simulink model "Lab2_AircraftEPS"  (Simulink 8.0)
settings: Solver=ode3  StartTime=0.0  StopTime=10  RelTol=1e-3
PreLoadFcn:
  | warning off
  | Ts=10e-6;
InitFcn:
  | warning off
  | Ts=10e-6;
undefined symbols (not defined in the file or in its folder): D1, Delta, sigbuilder_block
libraries: powerlib x91, sps_avr x4, powerlib_extras x4, checkVoltage x4
(part 2 of 2)

== system Lab2_AircraftEPS/TRU 28Vdc 4kW ==
  Ground1 : powerlib/Elements/Ground  LConnTagsString=a
  Ground2 : powerlib/Elements/Ground  LConnTagsString=a
  Ground4 : powerlib/Elements/Ground  LConnTagsString=a
  Series RLC Branch1 : powerlib/Elements/Series RLC Branch  LConnTagsString=__new0  RConnTagsString=__new0  BranchType=L  Resistance=[]  Inductance=2e-3  SetiL0=on  InitialCurrent=0  Capacitance=[]  Setx0=off  InitialVoltage=0  Measurements=Branch voltage and current
  Series RLC Branch2 : powerlib/Elements/Series RLC Branch  LConnTagsString=__new0  RConnTagsString=__new0  BranchType=C  Resistance=[]  Inductance=[]  SetiL0=off  InitialCurrent=0  Capacitance=1e-6  Setx0=off  InitialVoltage=0  Measurements=None
  Series RLC Branch4 : powerlib/Elements/Series RLC Branch  LConnTagsString=__new0  RConnTagsString=__new0  BranchType=L  Resistance=[]  Inductance=2e-3  SetiL0=off  InitialCurrent=0  Capacitance=[]  Setx0=off  InitialVoltage=0  Measurements=Branch voltage and current
  Three-Phase Transformer (Three Windings) : powerlib/Elements/Three-Phase Transformer (Three Windings)  Winding1Connection=Yn  UNITS=pu  NominalPower=[ 4200 , 400 ]  Winding1=[ 115 , 0.0002 , 0 ]  Winding2Connection=Delta (D1)  Winding2=[ 22 , 0.0002 , 0 ]  Winding3Connection=Delta (D1)  Winding3=[ 22 , 0.0002 , 0]  SetSaturation=off  Rm=500  Lm=500*10  Saturation=[ 0,0 ; 0.0024,1.2 ; 1.0,1.52 ]  Hysteresis=off  DataFile='hysteresis'  SetInitialFlux=off  InitialFluxes=[0.8 -0.8 0.7]  Measurements=None  MoreParameters=off  BreakLoop=off  DataType=off  TransfoNumber=0
  Universal Bridge : powerlib/Power Electronics/Universal Bridge  Arms=3  SnubberResistance=1e3  SnubberCapacitance=1e-6  Device=Diodes  Ron=1e-3  Lon=0  ForwardVoltages="[  0  0  ]"  ForwardVoltage=0.8  GTOparameters=[ 10e-6 , 20e-6 ]  IGBTparameters=[ 1e-6 , 2e-6 ]  Measurements=None  Measurements_2=None  converterType=Rectifier
  Universal Bridge1 : powerlib/Power Electronics/Universal Bridge  Arms=3  SnubberResistance=1e3  SnubberCapacitance=1e-6  Device=Diodes  Ron=1e-3  Lon=0  ForwardVoltages="[  0  0  ]"  ForwardVoltage=0.8  GTOparameters=[ 10e-6 , 20e-6 ]  IGBTparameters=[ 1e-6 , 2e-6 ]  Measurements=None  Measurements_2=None  converterType=Rectifier
  A : PMIOPort  Port=1  Side=Left
  B : PMIOPort  Port=2  Side=Left
  + : PMIOPort  Port=3  Side=Right
  C : PMIOPort  Port=4  Side=Left
  connections:
  Ground2/LConn1 -- Series RLC Branch2/RConn1
  Ground1/LConn1 -- Universal Bridge/RConn2 -- Universal Bridge1/RConn2
  Three-Phase Transformer (Three Windings)/RConn1 -- Universal Bridge/LConn1
  Three-Phase Transformer (Three Windings)/RConn2 -- Universal Bridge/LConn2
  Three-Phase Transformer (Three Windings)/RConn3 -- Universal Bridge/LConn3
  A/RConn1 -- Three-Phase Transformer (Three Windings)/LConn1
  B/RConn1 -- Three-Phase Transformer (Three Windings)/LConn2
  C/RConn1 -- Three-Phase Transformer (Three Windings)/LConn3
  Ground4/LConn1 -- Three-Phase Transformer (Three Windings)/LConn4
  Series RLC Branch1/LConn1 -- Universal Bridge/RConn1
  Series RLC Branch2/LConn1 -- Series RLC Branch1/RConn1 -- +/RConn1 -- Series RLC Branch4/LConn1
  Three-Phase Transformer (Three Windings)/RConn4 -- Universal Bridge1/LConn1
  Three-Phase Transformer (Three Windings)/RConn5 -- Universal Bridge1/LConn2
  Three-Phase Transformer (Three Windings)/RConn6 -- Universal Bridge1/LConn3
  Universal Bridge1/RConn1 -- Series RLC Branch4/RConn1

== system Lab2_AircraftEPS/TRU 28Vdc 4kW3 ==
  Ground1 : powerlib/Elements/Ground  LConnTagsString=a
  Ground2 : powerlib/Elements/Ground  LConnTagsString=a
  Ground4 : powerlib/Elements/Ground  LConnTagsString=a
  Series RLC Branch1 : powerlib/Elements/Series RLC Branch  LConnTagsString=__new0  RConnTagsString=__new0  BranchType=L  Resistance=[]  Inductance=2e-3  SetiL0=on  InitialCurrent=0  Capacitance=[]  Setx0=off  InitialVoltage=0  Measurements=Branch voltage and current
  Series RLC Branch2 : powerlib/Elements/Series RLC Branch  LConnTagsString=__new0  RConnTagsString=__new0  BranchType=C  Resistance=[]  Inductance=[]  SetiL0=off  InitialCurrent=0  Capacitance=1e-6  Setx0=off  InitialVoltage=0  Measurements=None
  Series RLC Branch4 : powerlib/Elements/Series RLC Branch  LConnTagsString=__new0  RConnTagsString=__new0  BranchType=L  Resistance=[]  Inductance=2e-3  SetiL0=off  InitialCurrent=0  Capacitance=[]  Setx0=off  InitialVoltage=0  Measurements=Branch voltage and current
  Three-Phase Transformer (Three Windings) : powerlib/Elements/Three-Phase Transformer (Three Windings)  Winding1Connection=Yn  UNITS=pu  NominalPower=[ 4200 , 400 ]  Winding1=[ 115 , 0.0002 , 0 ]  Winding2Connection=Delta (D1)  Winding2=[ 22 , 0.0002 , 0 ]  Winding3Connection=Delta (D1)  Winding3=[ 22 , 0.0002 , 0]  SetSaturation=off  Rm=500  Lm=500*10  Saturation=[ 0,0 ; 0.0024,1.2 ; 1.0,1.52 ]  Hysteresis=off  DataFile='hysteresis'  SetInitialFlux=off  InitialFluxes=[0.8 -0.8 0.7]  Measurements=None  MoreParameters=off  BreakLoop=off  DataType=off  TransfoNumber=0
  Universal Bridge : powerlib/Power Electronics/Universal Bridge  Arms=3  SnubberResistance=1e3  SnubberCapacitance=1e-6  Device=Diodes  Ron=1e-3  Lon=0  ForwardVoltages="[  0  0  ]"  ForwardVoltage=0.8  GTOparameters=[ 10e-6 , 20e-6 ]  IGBTparameters=[ 1e-6 , 2e-6 ]  Measurements=None  Measurements_2=None  converterType=Rectifier
  Universal Bridge1 : powerlib/Power Electronics/Universal Bridge  Arms=3  SnubberResistance=1e3  SnubberCapacitance=1e-6  Device=Diodes  Ron=1e-3  Lon=0  ForwardVoltages="[  0  0  ]"  ForwardVoltage=0.8  GTOparameters=[ 10e-6 , 20e-6 ]  IGBTparameters=[ 1e-6 , 2e-6 ]  Measurements=None  Measurements_2=None  converterType=Rectifier
  A : PMIOPort  Port=1  Side=Left
  B : PMIOPort  Port=2  Side=Left
  + : PMIOPort  Port=3  Side=Right
  C : PMIOPort  Port=4  Side=Left
  connections:
  Ground2/LConn1 -- Series RLC Branch2/RConn1
  Ground1/LConn1 -- Universal Bridge/RConn2 -- Universal Bridge1/RConn2
  Three-Phase Transformer (Three Windings)/RConn1 -- Universal Bridge/LConn1
  Three-Phase Transformer (Three Windings)/RConn2 -- Universal Bridge/LConn2
  Three-Phase Transformer (Three Windings)/RConn3 -- Universal Bridge/LConn3
  A/RConn1 -- Three-Phase Transformer (Three Windings)/LConn1
  B/RConn1 -- Three-Phase Transformer (Three Windings)/LConn2
  C/RConn1 -- Three-Phase Transformer (Three Windings)/LConn3
  Ground4/LConn1 -- Three-Phase Transformer (Three Windings)/LConn4
  Series RLC Branch1/LConn1 -- Universal Bridge/RConn1
  Series RLC Branch2/LConn1 -- Series RLC Branch1/RConn1 -- +/RConn1 -- Series RLC Branch4/LConn1
  Three-Phase Transformer (Three Windings)/RConn4 -- Universal Bridge1/LConn1
  Three-Phase Transformer (Three Windings)/RConn5 -- Universal Bridge1/LConn2
  Three-Phase Transformer (Three Windings)/RConn6 -- Universal Bridge1/LConn3
  Universal Bridge1/RConn1 -- Series RLC Branch4/RConn1

== system Lab2_AircraftEPS/APU1/Fault Contactor ==
  Fault : Inport
  In1 : Inport  Port=2
  Constant : Constant  Value=0
  Switch : Switch  Threshold=0.5
  out : Outport
  wires:
  Fault/1 -> Switch/2
  Constant/1 -> Switch/3
  In1/1 -> Switch/1
  Switch/1 -> out/1

== system Lab2_AircraftEPS/APU1/Feedback measurements &  main contactor ==
  note: Primary Distribution
  GLC control : Inport
  Contactor : Subsystem
  P.O.R  and CTA : powerlib/Measurements/Three-Phase V-I Measurement  VoltageMeasurement=phase-to-phase  SetLabelV=off  LabelV=Vabc  Vpu=off  VpuLL=off  CurrentMeasurement=yes  SetLabelI=off  LabelI=Iabc  Ipu=off  Pbase=100e6  Vbase=500e3  OutputType=Complex  PhasorSimulation=off  PSBequivalent=0
  parasitic resistive load : powerlib/Elements/Three-Phase Series RLC Load  LConnTagsString=A|B|C  Configuration=Y (grounded)  NominalVoltage=115  NominalFrequency=400  ActivePower=5000  InductivePower=0  CapacitivePower=0  Measurements=None  LoadType=constant Z
  in_a : PMIOPort  Port=1  Side=Left
  in_b : PMIOPort  Port=2  Side=Left
  in_c : PMIOPort  Port=3  Side=Left
  out_a : PMIOPort  Port=4  Side=Right
  out_b : PMIOPort  Port=5  Side=Right
  out_c : PMIOPort  Port=6  Side=Right
  Vabc : Outport
  Iabc : Outport  Port=2
  wires:
  GLC control/1 -> Contactor/1(com)
  P.O.R  and CTA/1 -> Vabc/1
  P.O.R  and CTA/2 -> Iabc/1
  connections:
  in_a/RConn1 -- P.O.R  and CTA/LConn1 -- parasitic resistive load/LConn1
  in_b/RConn1 -- P.O.R  and CTA/LConn2 -- parasitic resistive load/LConn2
  in_c/RConn1 -- P.O.R  and CTA/LConn3 -- parasitic resistive load/LConn3
  P.O.R  and CTA/RConn1 -- Contactor/LConn1
  P.O.R  and CTA/RConn2 -- Contactor/LConn2
  P.O.R  and CTA/RConn3 -- Contactor/LConn3
  Contactor/RConn1 -- out_a/RConn1
  out_b/RConn1 -- Contactor/RConn2
  Contactor/RConn3 -- out_c/RConn1

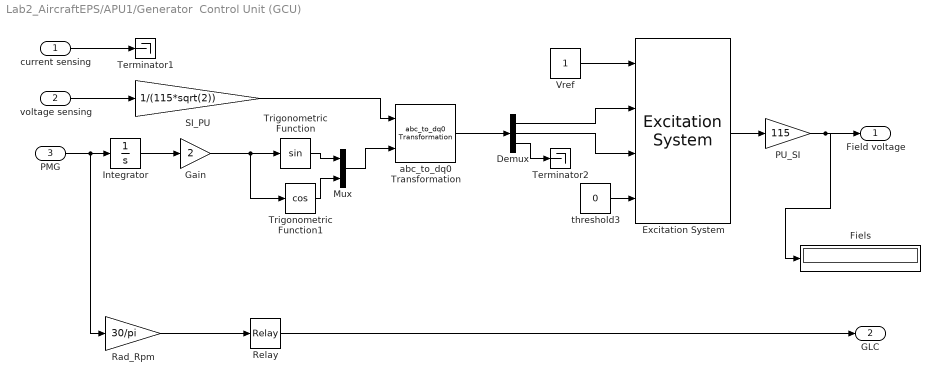
== system Lab2_AircraftEPS/APU1/Generator  Control Unit (GCU) ==
  current sensing : Inport
  voltage sensing : Inport  Port=2
  PMG : Inport  Port=3
  Demux : Demux  Outputs=3
  Excitation System : sps_avr/Excitation System   tr=20e-3  reg=[ 300, 0.001 ]  exc=[ 1, 0 ]  tgr=[ 0, 0 ]  damp=[ 0.001, 0.1 ]  sat=[ 0, 0 ]  lim=[ -2, 2, 0 ]  v0=[1 0]
  Fiels : Display
      settings: SampleTime=1e-2
  Gain : Gain  Gain=2
  Integrator : Integrator
  Mux : Mux  Inputs=2
  PU_SI : Gain  Gain=115
  Rad_Rpm : Gain  Gain=30/pi
  Relay : Relay  OnSwitchValue=9000  OffSwitchValue=8900
  SI_PU : Gain  Gain=1/(115*sqrt(2))
  Terminator1 : Terminator
  Terminator2 : Terminator
  Trigonometric Function : Trigonometry
  Trigonometric Function1 : Trigonometry  Operator=cos
  Vref : Constant
  abc_to_dq0 Transformation : powerlib_extras/Measurements/abc_to_dq0 Transformation
  threshold3 : Constant  Value=0
  Field voltage : Outport
  GLC : Outport  Port=2
  wires:
  Relay/1 -> GLC/1
  Demux/3 -> Terminator2/1
  current sensing/1 -> Terminator1/1
  threshold3/1 -> Excitation System/4
  Vref/1 -> Excitation System/1
  Rad_Rpm/1 -> Relay/1
  PU_SI/1 -> Field voltage/1, Fiels/1
  Excitation System/1 -> PU_SI/1
  SI_PU/1 -> abc_to_dq0 Transformation/1
  Demux/2 -> Excitation System/3
  Demux/1 -> Excitation System/2
  abc_to_dq0 Transformation/1 -> Demux/1
  Mux/1 -> abc_to_dq0 Transformation/2
  Trigonometric Function1/1 -> Mux/2
  Trigonometric Function/1 -> Mux/1
  Gain/1 -> Trigonometric Function1/1, Trigonometric Function/1
  Integrator/1 -> Gain/1
  voltage sensing/1 -> SI_PU/1
  PMG/1 -> Rad_Rpm/1, Integrator/1

== system Lab2_AircraftEPS/APU1/Mechanical engine (turbine) ==
  Demux : Demux  Tag=STV Demux  Outputs=1
  FromWs : FromWorkspace  Tag=STV FromWs  VariableName=tuvar  SampleTime=0  SigBuilderData=DataTag0  VnvData=DataTag1
      SigBuilderData=|
      | common.afterFinalStr = 'Extrapolate'
      | common.sampleTime = 0
      | dataSet.timeRange = [0 10]
      | dataSet.name = 'Group 1'
      | sbobj.Groups.Name = 'Group 1'
      | sbobj.Groups.Signals.Name = 'Signal 1'
      | sbobj.Groups.Signals.XData = [0 0.2 0.4 0.5 1 2 3 4.5 6 10]
      | sbobj.Groups.Signals.YData = [15000 15000 15000 15000 15000 15000 15000 15000 15000 15000]
  Signal 1 : Outport  Tag=STV Outport
  wires:
  FromWs/1 -> Demux/1
  Demux/1 -> Signal 1/1

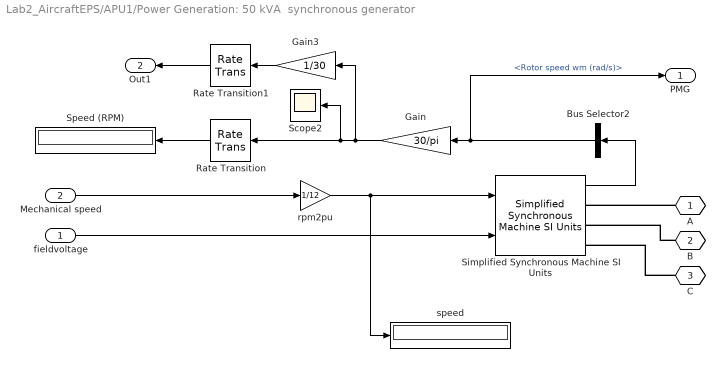
== system Lab2_AircraftEPS/APU1/Power Generation: 50 kVA  synchronous generator ==
  fieldvoltage : Inport
  Mechanical speed : Inport  Port=2
  Bus Selector2 : BusSelector  OutputSignals=Rotor speed wm (rad/s)
  Gain : Gain  Gain=30/pi
  Gain3 : Gain  Gain=1/30
  Rate Transition : RateTransition  OutPortSampleTimeOpt=Inherit  OutPortSampleTime=Ts
  Rate Transition1 : RateTransition  OutPortSampleTimeOpt=Inherit  OutPortSampleTime=Ts
  Scope2 : Scope
      settings: TimeRange=1  YMin=13545  YMax=13575  SaveName=ScopeData3  Decimation=100  SampleTime=1e-3
  Simplified Synchronous Machine SI Units : powerlib/Machines/Simplified Synchronous Machine SI Units  ConnectionType=3-wire Y  MechanicalLoad=Speed w  NominalParameters=[50e3 115 400]  Mechanical=[0.02 0 2]  InternalRL="[0.0204  0.08104e-3]"  InitialConditions=[-99,0 0,0,0 0,0,0]  Units=1  LoadFlowParameters=[1 0 0 0 0]  TsPowergui=0  TsBlock=-1  BusType=PV  Pref=0  Qref=0  Qmin=-inf  Qmax=+inf  PLF=0  QLF=0
  Speed (RPM) : Display
      settings: SampleTime=1e-2
  rpm2pu : Gain  Gain=1/12
  speed : Display
      settings: SampleTime=1e-2
  A : PMIOPort  Tag=PMCPort  Port=1  Side=Right
  B : PMIOPort  Tag=PMCPort  Port=2  Side=Right
  C : PMIOPort  Tag=PMCPort  Port=3  Side=Right
  PMG : Outport
  Out1 : Outport  Port=2
  wires:
  Simplified Synchronous Machine SI Units/1 -> Bus Selector2/1
  fieldvoltage/1 -> Simplified Synchronous Machine SI Units/2
  Bus Selector2/1 -> Gain/1, PMG/1  "<Rotor speed wm (rad/s)>"
  Gain/1 -> Gain3/1, Scope2/1, Rate Transition/1
  Gain3/1 -> Rate Transition1/1
  Mechanical speed/1 -> rpm2pu/1
  rpm2pu/1 -> Simplified Synchronous Machine SI Units/1, speed/1
  Rate Transition/1 -> Speed (RPM)/1
  Rate Transition1/1 -> Out1/1
  connections:
  A/RConn1 -- Simplified Synchronous Machine SI Units/RConn1
  B/RConn1 -- Simplified Synchronous Machine SI Units/RConn2
  C/RConn1 -- Simplified Synchronous Machine SI Units/RConn3

== system Lab2_AircraftEPS/APU1/Sensor ==
  Three Phase  Measurement : powerlib/Measurements/Three-Phase V-I Measurement  VoltageMeasurement=phase-to-phase  SetLabelV=off  LabelV=Vabc  Vpu=off  VpuLL=off  CurrentMeasurement=yes  SetLabelI=off  LabelI=Iabc  Ipu=off  Pbase=100e6  Vbase=500e3  OutputType=Complex  PhasorSimulation=off  PSBequivalent=0
  parasitic  load : powerlib/Elements/Three-Phase Series RLC Load  LConnTagsString=A|B|C  Configuration=Y (grounded)  NominalVoltage=115  NominalFrequency=400  ActivePower=5000  InductivePower=0  CapacitivePower=0  Measurements=None  LoadType=constant Z
  A : PMIOPort  Port=1  Side=Left
  B : PMIOPort  Port=2  Side=Left
  a : PMIOPort  Port=3  Side=Right
  b : PMIOPort  Port=4  Side=Right
  C : PMIOPort  Port=5  Side=Left
  c : PMIOPort  Port=6  Side=Right
  Vabc : Outport
  Iabc : Outport  Port=2
  wires:
  Three Phase  Measurement/1 -> Vabc/1
  Three Phase  Measurement/2 -> Iabc/1
  connections:
  A/RConn1 -- Three Phase  Measurement/LConn1 -- parasitic  load/LConn1
  B/RConn1 -- Three Phase  Measurement/LConn2 -- parasitic  load/LConn2
  C/RConn1 -- Three Phase  Measurement/LConn3 -- parasitic  load/LConn3
  a/RConn1 -- Three Phase  Measurement/RConn1
  b/RConn1 -- Three Phase  Measurement/RConn2
  c/RConn1 -- Three Phase  Measurement/RConn3

== system Lab2_AircraftEPS/APU2/Fault Contactor ==
  Fault : Inport
  In1 : Inport  Port=2
  Constant : Constant  Value=0
  Switch : Switch  Threshold=0.5
  out : Outport
  wires:
  Fault/1 -> Switch/2
  Constant/1 -> Switch/3
  In1/1 -> Switch/1
  Switch/1 -> out/1

== system Lab2_AircraftEPS/APU2/Feedback measurements &  main contactor ==
  note: Primary Distribution
  GLC control : Inport
  Contactor : Subsystem
  P.O.R  and CTA : powerlib/Measurements/Three-Phase V-I Measurement  VoltageMeasurement=phase-to-phase  SetLabelV=off  LabelV=Vabc  Vpu=off  VpuLL=off  CurrentMeasurement=yes  SetLabelI=off  LabelI=Iabc  Ipu=off  Pbase=100e6  Vbase=500e3  OutputType=Complex  PhasorSimulation=off  PSBequivalent=0
  parasitic resistive load : powerlib/Elements/Three-Phase Series RLC Load  LConnTagsString=A|B|C  Configuration=Y (grounded)  NominalVoltage=200  NominalFrequency=400  ActivePower=5000  InductivePower=0  CapacitivePower=0  Measurements=None  LoadType=constant Z
  in_a : PMIOPort  Port=1  Side=Left
  in_b : PMIOPort  Port=2  Side=Left
  in_c : PMIOPort  Port=3  Side=Left
  out_a : PMIOPort  Port=4  Side=Right
  out_b : PMIOPort  Port=5  Side=Right
  out_c : PMIOPort  Port=6  Side=Right
  Vabc : Outport
  Iabc : Outport  Port=2
  wires:
  GLC control/1 -> Contactor/1(com)
  P.O.R  and CTA/1 -> Vabc/1
  P.O.R  and CTA/2 -> Iabc/1
  connections:
  in_a/RConn1 -- P.O.R  and CTA/LConn1 -- parasitic resistive load/LConn1
  in_b/RConn1 -- P.O.R  and CTA/LConn2 -- parasitic resistive load/LConn2
  in_c/RConn1 -- P.O.R  and CTA/LConn3 -- parasitic resistive load/LConn3
  P.O.R  and CTA/RConn1 -- Contactor/LConn1
  P.O.R  and CTA/RConn2 -- Contactor/LConn2
  P.O.R  and CTA/RConn3 -- Contactor/LConn3
  Contactor/RConn1 -- out_a/RConn1
  out_b/RConn1 -- Contactor/RConn2
  Contactor/RConn3 -- out_c/RConn1

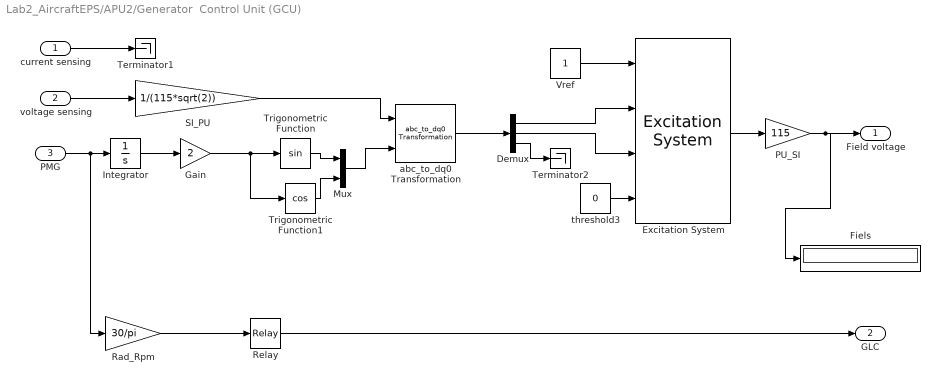
== system Lab2_AircraftEPS/APU2/Generator  Control Unit (GCU) ==
  current sensing : Inport
  voltage sensing : Inport  Port=2
  PMG : Inport  Port=3
  Demux : Demux  Outputs=3
  Excitation System : sps_avr/Excitation System   tr=20e-3  reg=[ 300, 0.001 ]  exc=[ 1, 0 ]  tgr=[ 0, 0 ]  damp=[ 0.001, 0.1 ]  sat=[ 0, 0 ]  lim=[ -2, 2, 0 ]  v0=[1 0]
  Fiels : Display
      settings: SampleTime=1e-2
  Gain : Gain  Gain=2
  Integrator : Integrator
  Mux : Mux  Inputs=2
  PU_SI : Gain  Gain=115
  Rad_Rpm : Gain  Gain=30/pi
  Relay : Relay  OnSwitchValue=9000  OffSwitchValue=8900
  SI_PU : Gain  Gain=1/(115*sqrt(2))
  Terminator1 : Terminator
  Terminator2 : Terminator
  Trigonometric Function : Trigonometry
  Trigonometric Function1 : Trigonometry  Operator=cos
  Vref : Constant
  abc_to_dq0 Transformation : powerlib_extras/Measurements/abc_to_dq0 Transformation
  threshold3 : Constant  Value=0
  Field voltage : Outport
  GLC : Outport  Port=2
  wires:
  Relay/1 -> GLC/1
  Demux/3 -> Terminator2/1
  current sensing/1 -> Terminator1/1
  threshold3/1 -> Excitation System/4
  Vref/1 -> Excitation System/1
  Rad_Rpm/1 -> Relay/1
  PU_SI/1 -> Field voltage/1, Fiels/1
  Excitation System/1 -> PU_SI/1
  SI_PU/1 -> abc_to_dq0 Transformation/1
  Demux/2 -> Excitation System/3
  Demux/1 -> Excitation System/2
  abc_to_dq0 Transformation/1 -> Demux/1
  Mux/1 -> abc_to_dq0 Transformation/2
  Trigonometric Function1/1 -> Mux/2
  Trigonometric Function/1 -> Mux/1
  Gain/1 -> Trigonometric Function1/1, Trigonometric Function/1
  Integrator/1 -> Gain/1
  voltage sensing/1 -> SI_PU/1
  PMG/1 -> Rad_Rpm/1, Integrator/1

== system Lab2_AircraftEPS/APU2/Mechanical engine (turbine) ==
  Demux : Demux  Tag=STV Demux  Outputs=1
  FromWs : FromWorkspace  Tag=STV FromWs  VariableName=tuvar  SampleTime=0  SigBuilderData=DataTag2  VnvData=DataTag3
      SigBuilderData=|
      | common.afterFinalStr = 'Extrapolate'
      | common.sampleTime = 0
      | dataSet.timeRange = [0 10]
      | dataSet.name = 'Group 1'
      | sbobj.Groups.Name = 'Group 1'
      | sbobj.Groups.Signals.Name = 'Signal 1'
      | sbobj.Groups.Signals.XData = [0 0.2 0.4 0.5 1 2 3 4.5 6 10]
      | sbobj.Groups.Signals.YData = [15000 15000 15000 15000 15000 15000 15000 15000 15000 15000]
  Signal 1 : Outport  Tag=STV Outport
  wires:
  FromWs/1 -> Demux/1
  Demux/1 -> Signal 1/1

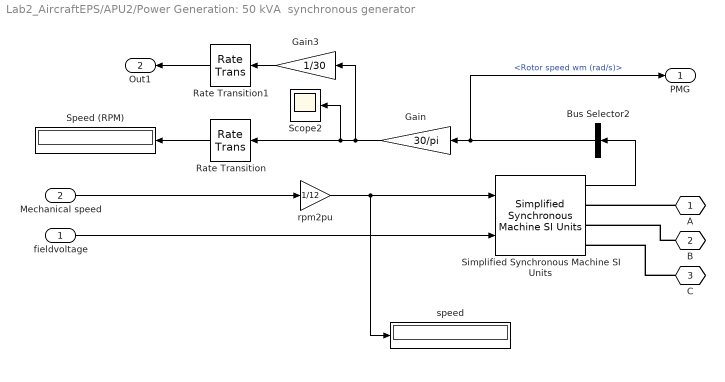
== system Lab2_AircraftEPS/APU2/Power Generation: 50 kVA  synchronous generator ==
  fieldvoltage : Inport
  Mechanical speed : Inport  Port=2
  Bus Selector2 : BusSelector  OutputSignals=Rotor speed wm (rad/s)
  Gain : Gain  Gain=30/pi
  Gain3 : Gain  Gain=1/30
  Rate Transition : RateTransition  OutPortSampleTimeOpt=Inherit  OutPortSampleTime=Ts
  Rate Transition1 : RateTransition  OutPortSampleTimeOpt=Inherit  OutPortSampleTime=Ts
  Scope2 : Scope
      settings: TimeRange=1  YMin=13545  YMax=13575  SaveName=ScopeData3  Decimation=100  SampleTime=1e-3
  Simplified Synchronous Machine SI Units : powerlib/Machines/Simplified Synchronous Machine SI Units  ConnectionType=3-wire Y  MechanicalLoad=Speed w  NominalParameters=[50e3 115 400]  Mechanical=[0.02 0 2]  InternalRL="[0.0204  0.08104e-3]"  InitialConditions=[-99,0 0,0,0 0,0,0]  Units=1  LoadFlowParameters=[1 0 0 0 0]  TsPowergui=0  TsBlock=-1  BusType=PV  Pref=0  Qref=0  Qmin=-inf  Qmax=+inf  PLF=0  QLF=0
  Speed (RPM) : Display
      settings: SampleTime=1e-2
  rpm2pu : Gain  Gain=1/12
  speed : Display
      settings: SampleTime=1e-2
  A : PMIOPort  Tag=PMCPort  Port=1  Side=Right
  B : PMIOPort  Tag=PMCPort  Port=2  Side=Right
  C : PMIOPort  Tag=PMCPort  Port=3  Side=Right
  PMG : Outport
  Out1 : Outport  Port=2
  wires:
  Simplified Synchronous Machine SI Units/1 -> Bus Selector2/1
  fieldvoltage/1 -> Simplified Synchronous Machine SI Units/2
  Bus Selector2/1 -> Gain/1, PMG/1  "<Rotor speed wm (rad/s)>"
  Gain/1 -> Gain3/1, Scope2/1, Rate Transition/1
  Gain3/1 -> Rate Transition1/1
  Mechanical speed/1 -> rpm2pu/1
  rpm2pu/1 -> Simplified Synchronous Machine SI Units/1, speed/1
  Rate Transition/1 -> Speed (RPM)/1
  Rate Transition1/1 -> Out1/1
  connections:
  A/RConn1 -- Simplified Synchronous Machine SI Units/RConn1
  B/RConn1 -- Simplified Synchronous Machine SI Units/RConn2
  C/RConn1 -- Simplified Synchronous Machine SI Units/RConn3

== system Lab2_AircraftEPS/APU2/Sensor ==
  Three Phase  Measurement : powerlib/Measurements/Three-Phase V-I Measurement  VoltageMeasurement=phase-to-phase  SetLabelV=off  LabelV=Vabc  Vpu=off  VpuLL=off  CurrentMeasurement=yes  SetLabelI=off  LabelI=Iabc  Ipu=off  Pbase=100e6  Vbase=500e3  OutputType=Complex  PhasorSimulation=off  PSBequivalent=0
  parasitic  load : powerlib/Elements/Three-Phase Series RLC Load  LConnTagsString=A|B|C  Configuration=Y (grounded)  NominalVoltage=115  NominalFrequency=400  ActivePower=5000  InductivePower=0  CapacitivePower=0  Measurements=None  LoadType=constant Z
  A : PMIOPort  Port=1  Side=Left
  B : PMIOPort  Port=2  Side=Left
  a : PMIOPort  Port=3  Side=Right
  b : PMIOPort  Port=4  Side=Right
  C : PMIOPort  Port=5  Side=Left
  c : PMIOPort  Port=6  Side=Right
  Vabc : Outport
  Iabc : Outport  Port=2
  wires:
  Three Phase  Measurement/1 -> Vabc/1
  Three Phase  Measurement/2 -> Iabc/1
  connections:
  A/RConn1 -- Three Phase  Measurement/LConn1 -- parasitic  load/LConn1
  B/RConn1 -- Three Phase  Measurement/LConn2 -- parasitic  load/LConn2
  C/RConn1 -- Three Phase  Measurement/LConn3 -- parasitic  load/LConn3
  a/RConn1 -- Three Phase  Measurement/RConn1
  b/RConn1 -- Three Phase  Measurement/RConn2
  c/RConn1 -- Three Phase  Measurement/RConn3

== system Lab2_AircraftEPS/B1/Contactor ==
  com : Inport
  Ideal Switch : powerlib/Power Electronics/Ideal Switch  Ron=0.001  Lon=0  IC=0  Rs=1e3  Cs=inf  Measurements=off
  Ideal Switch1 : powerlib/Power Electronics/Ideal Switch  Ron=0.001  Lon=0  IC=0  Rs=1e3  Cs=inf  Measurements=off
  Ideal Switch2 : powerlib/Power Electronics/Ideal Switch  Ron=0.001  Lon=0  IC=0  Rs=1e3  Cs=inf  Measurements=off
  A : PMIOPort  Port=1  Side=Left
  a : PMIOPort  Port=2  Side=Right
  B : PMIOPort  Port=3  Side=Left
  b : PMIOPort  Port=4  Side=Right
  C : PMIOPort  Port=5  Side=Left
  c : PMIOPort  Port=6  Side=Right
  wires:
  com/1 -> Ideal Switch/1, Ideal Switch2/1, Ideal Switch1/1
  connections:
  A/RConn1 -- Ideal Switch/LConn1
  a/RConn1 -- Ideal Switch/RConn1
  B/RConn1 -- Ideal Switch1/LConn1
  b/RConn1 -- Ideal Switch1/RConn1
  C/RConn1 -- Ideal Switch2/LConn1
  c/RConn1 -- Ideal Switch2/RConn1

== system Lab2_AircraftEPS/B10/Contactor ==
  com : Inport
  Ideal Switch : powerlib/Power Electronics/Ideal Switch  Ron=0.001  Lon=0  IC=0  Rs=1e3  Cs=inf  Measurements=off
  A : PMIOPort  Port=1  Side=Left
  a : PMIOPort  Port=2  Side=Right
  wires:
  com/1 -> Ideal Switch/1
  connections:
  A/RConn1 -- Ideal Switch/LConn1
  a/RConn1 -- Ideal Switch/RConn1

== system Lab2_AircraftEPS/B11/Contactor ==
  com : Inport
  Ideal Switch : powerlib/Power Electronics/Ideal Switch  Ron=0.001  Lon=0  IC=0  Rs=1e3  Cs=inf  Measurements=off
  A : PMIOPort  Port=1  Side=Left
  a : PMIOPort  Port=2  Side=Right
  wires:
  com/1 -> Ideal Switch/1
  connections:
  A/RConn1 -- Ideal Switch/LConn1
  a/RConn1 -- Ideal Switch/RConn1

== system Lab2_AircraftEPS/B12/Contactor ==
  com : Inport
  Ideal Switch : powerlib/Power Electronics/Ideal Switch  Ron=0.001  Lon=0  IC=0  Rs=1e3  Cs=inf  Measurements=off
  A : PMIOPort  Port=1  Side=Left
  a : PMIOPort  Port=2  Side=Right
  wires:
  com/1 -> Ideal Switch/1
  connections:
  A/RConn1 -- Ideal Switch/LConn1
  a/RConn1 -- Ideal Switch/RConn1

== system Lab2_AircraftEPS/B2/Contactor ==
  com : Inport
  Ideal Switch : powerlib/Power Electronics/Ideal Switch  Ron=0.001  Lon=0  IC=0  Rs=1e3  Cs=inf  Measurements=off
  Ideal Switch1 : powerlib/Power Electronics/Ideal Switch  Ron=0.001  Lon=0  IC=0  Rs=1e3  Cs=inf  Measurements=off
  Ideal Switch2 : powerlib/Power Electronics/Ideal Switch  Ron=0.001  Lon=0  IC=0  Rs=1e3  Cs=inf  Measurements=off
  A : PMIOPort  Port=1  Side=Left
  a : PMIOPort  Port=2  Side=Right
  B : PMIOPort  Port=3  Side=Left
  b : PMIOPort  Port=4  Side=Right
  C : PMIOPort  Port=5  Side=Left
  c : PMIOPort  Port=6  Side=Right
  wires:
  com/1 -> Ideal Switch/1, Ideal Switch2/1, Ideal Switch1/1
  connections:
  A/RConn1 -- Ideal Switch/LConn1
  a/RConn1 -- Ideal Switch/RConn1
  B/RConn1 -- Ideal Switch1/LConn1
  b/RConn1 -- Ideal Switch1/RConn1
  C/RConn1 -- Ideal Switch2/LConn1
  c/RConn1 -- Ideal Switch2/RConn1

== system Lab2_AircraftEPS/B3/Contactor ==
  com : Inport
  Ideal Switch : powerlib/Power Electronics/Ideal Switch  Ron=0.001  Lon=0  IC=0  Rs=1e3  Cs=inf  Measurements=off
  Ideal Switch1 : powerlib/Power Electronics/Ideal Switch  Ron=0.001  Lon=0  IC=0  Rs=1e3  Cs=inf  Measurements=off
  Ideal Switch2 : powerlib/Power Electronics/Ideal Switch  Ron=0.001  Lon=0  IC=0  Rs=1e3  Cs=inf  Measurements=off
  A : PMIOPort  Port=1  Side=Left
  a : PMIOPort  Port=2  Side=Right
  B : PMIOPort  Port=3  Side=Left
  b : PMIOPort  Port=4  Side=Right
  C : PMIOPort  Port=5  Side=Left
  c : PMIOPort  Port=6  Side=Right
  wires:
  com/1 -> Ideal Switch/1, Ideal Switch2/1, Ideal Switch1/1
  connections:
  A/RConn1 -- Ideal Switch/LConn1
  a/RConn1 -- Ideal Switch/RConn1
  B/RConn1 -- Ideal Switch1/LConn1
  b/RConn1 -- Ideal Switch1/RConn1
  C/RConn1 -- Ideal Switch2/LConn1
  c/RConn1 -- Ideal Switch2/RConn1

== system Lab2_AircraftEPS/B4/Contactor ==
  com : Inport
  Ideal Switch : powerlib/Power Electronics/Ideal Switch  Ron=0.001  Lon=0  IC=0  Rs=1e3  Cs=inf  Measurements=off
  Ideal Switch1 : powerlib/Power Electronics/Ideal Switch  Ron=0.001  Lon=0  IC=0  Rs=1e3  Cs=inf  Measurements=off
  Ideal Switch2 : powerlib/Power Electronics/Ideal Switch  Ron=0.001  Lon=0  IC=0  Rs=1e3  Cs=inf  Measurements=off
  A : PMIOPort  Port=1  Side=Left
  a : PMIOPort  Port=2  Side=Right
  B : PMIOPort  Port=3  Side=Left
  b : PMIOPort  Port=4  Side=Right
  C : PMIOPort  Port=5  Side=Left
  c : PMIOPort  Port=6  Side=Right
  wires:
  com/1 -> Ideal Switch/1, Ideal Switch2/1, Ideal Switch1/1
  connections:
  A/RConn1 -- Ideal Switch/LConn1
  a/RConn1 -- Ideal Switch/RConn1
  B/RConn1 -- Ideal Switch1/LConn1
  b/RConn1 -- Ideal Switch1/RConn1
  C/RConn1 -- Ideal Switch2/LConn1
  c/RConn1 -- Ideal Switch2/RConn1

== system Lab2_AircraftEPS/B5/Contactor ==
  com : Inport
  Ideal Switch : powerlib/Power Electronics/Ideal Switch  Ron=0.001  Lon=0  IC=0  Rs=1e3  Cs=inf  Measurements=off
  Ideal Switch1 : powerlib/Power Electronics/Ideal Switch  Ron=0.001  Lon=0  IC=0  Rs=1e3  Cs=inf  Measurements=off
  Ideal Switch2 : powerlib/Power Electronics/Ideal Switch  Ron=0.001  Lon=0  IC=0  Rs=1e3  Cs=inf  Measurements=off
  A : PMIOPort  Port=1  Side=Left
  a : PMIOPort  Port=2  Side=Right
  B : PMIOPort  Port=3  Side=Left
  b : PMIOPort  Port=4  Side=Right
  C : PMIOPort  Port=5  Side=Left
  c : PMIOPort  Port=6  Side=Right
  wires:
  com/1 -> Ideal Switch/1, Ideal Switch2/1, Ideal Switch1/1
  connections:
  A/RConn1 -- Ideal Switch/LConn1
  a/RConn1 -- Ideal Switch/RConn1
  B/RConn1 -- Ideal Switch1/LConn1
  b/RConn1 -- Ideal Switch1/RConn1
  C/RConn1 -- Ideal Switch2/LConn1
  c/RConn1 -- Ideal Switch2/RConn1

== system Lab2_AircraftEPS/B6/Contactor ==
  com : Inport
  Ideal Switch : powerlib/Power Electronics/Ideal Switch  Ron=0.001  Lon=0  IC=0  Rs=1e3  Cs=inf  Measurements=off
  Ideal Switch1 : powerlib/Power Electronics/Ideal Switch  Ron=0.001  Lon=0  IC=0  Rs=1e3  Cs=inf  Measurements=off
  Ideal Switch2 : powerlib/Power Electronics/Ideal Switch  Ron=0.001  Lon=0  IC=0  Rs=1e3  Cs=inf  Measurements=off
  A : PMIOPort  Port=1  Side=Left
  a : PMIOPort  Port=2  Side=Right
  B : PMIOPort  Port=3  Side=Left
  b : PMIOPort  Port=4  Side=Right
  C : PMIOPort  Port=5  Side=Left
  c : PMIOPort  Port=6  Side=Right
  wires:
  com/1 -> Ideal Switch/1, Ideal Switch2/1, Ideal Switch1/1
  connections:
  A/RConn1 -- Ideal Switch/LConn1
  a/RConn1 -- Ideal Switch/RConn1
  B/RConn1 -- Ideal Switch1/LConn1
  b/RConn1 -- Ideal Switch1/RConn1
  C/RConn1 -- Ideal Switch2/LConn1
  c/RConn1 -- Ideal Switch2/RConn1

== system Lab2_AircraftEPS/B7/Contactor ==
  com : Inport
  Ideal Switch : powerlib/Power Electronics/Ideal Switch  Ron=0.001  Lon=0  IC=0  Rs=1e3  Cs=inf  Measurements=off
  Ideal Switch1 : powerlib/Power Electronics/Ideal Switch  Ron=0.001  Lon=0  IC=0  Rs=1e3  Cs=inf  Measurements=off
  Ideal Switch2 : powerlib/Power Electronics/Ideal Switch  Ron=0.001  Lon=0  IC=0  Rs=1e3  Cs=inf  Measurements=off
  A : PMIOPort  Port=1  Side=Left
  a : PMIOPort  Port=2  Side=Right
  B : PMIOPort  Port=3  Side=Left
  b : PMIOPort  Port=4  Side=Right
  C : PMIOPort  Port=5  Side=Left
  c : PMIOPort  Port=6  Side=Right
  wires:
  com/1 -> Ideal Switch/1, Ideal Switch2/1, Ideal Switch1/1
  connections:
  A/RConn1 -- Ideal Switch/LConn1
  a/RConn1 -- Ideal Switch/RConn1
  B/RConn1 -- Ideal Switch1/LConn1
  b/RConn1 -- Ideal Switch1/RConn1
  C/RConn1 -- Ideal Switch2/LConn1
  c/RConn1 -- Ideal Switch2/RConn1

== system Lab2_AircraftEPS/B8/Contactor ==
  com : Inport
  Ideal Switch : powerlib/Power Electronics/Ideal Switch  Ron=0.001  Lon=0  IC=0  Rs=1e3  Cs=inf  Measurements=off
  Ideal Switch1 : powerlib/Power Electronics/Ideal Switch  Ron=0.001  Lon=0  IC=0  Rs=1e3  Cs=inf  Measurements=off
  Ideal Switch2 : powerlib/Power Electronics/Ideal Switch  Ron=0.001  Lon=0  IC=0  Rs=1e3  Cs=inf  Measurements=off
  A : PMIOPort  Port=1  Side=Left
  a : PMIOPort  Port=2  Side=Right
  B : PMIOPort  Port=3  Side=Left
  b : PMIOPort  Port=4  Side=Right
  C : PMIOPort  Port=5  Side=Left
  c : PMIOPort  Port=6  Side=Right
  wires:
  com/1 -> Ideal Switch/1, Ideal Switch2/1, Ideal Switch1/1
  connections:
  A/RConn1 -- Ideal Switch/LConn1
  a/RConn1 -- Ideal Switch/RConn1
  B/RConn1 -- Ideal Switch1/LConn1
  b/RConn1 -- Ideal Switch1/RConn1
  C/RConn1 -- Ideal Switch2/LConn1
  c/RConn1 -- Ideal Switch2/RConn1

== system Lab2_AircraftEPS/B9/Contactor ==
  com : Inport
  Ideal Switch : powerlib/Power Electronics/Ideal Switch  Ron=0.001  Lon=0  IC=0  Rs=1e3  Cs=inf  Measurements=off
  A : PMIOPort  Port=1  Side=Left
  a : PMIOPort  Port=2  Side=Right
  wires:
  com/1 -> Ideal Switch/1
  connections:
  A/RConn1 -- Ideal Switch/LConn1
  a/RConn1 -- Ideal Switch/RConn1

== system Lab2_AircraftEPS/BPCU/UNUSED -  Load Management ==
  Constant : Constant
  Constant1 : Constant  Value=0
  B7 : Outport
  B8 : Outport  Port=2
  B9 : Outport  Port=3
  B10 : Outport  Port=4
  B11 : Outport  Port=5
  B12 : Outport  Port=6
  wires:
  Constant/1 -> B10/1, B9/1, B8/1, B7/1
  Constant1/1 -> B11/1, B12/1

== system Lab2_AircraftEPS/Left Engine HV/Fault Contactor ==
  Fault : Inport
  In1 : Inport  Port=2
  Constant : Constant  Value=0
  Switch : Switch  Threshold=0.5
  out : Outport
  wires:
  Fault/1 -> Switch/2
  Constant/1 -> Switch/3
  In1/1 -> Switch/1
  Switch/1 -> out/1

== system Lab2_AircraftEPS/Left Engine HV/Feedback measurements &  main contactor ==
  note: Primary Distribution
  GLC control : Inport
  Contactor : Subsystem
  P.O.R  and CTA : powerlib/Measurements/Three-Phase V-I Measurement  VoltageMeasurement=phase-to-phase  SetLabelV=off  LabelV=Vabc  Vpu=off  VpuLL=off  CurrentMeasurement=yes  SetLabelI=off  LabelI=Iabc  Ipu=off  Pbase=100e6  Vbase=500e3  OutputType=Complex  PhasorSimulation=off  PSBequivalent=0
  parasitic resistive load : powerlib/Elements/Three-Phase Series RLC Load  LConnTagsString=A|B|C  Configuration=Y (grounded)  NominalVoltage=115  NominalFrequency=400  ActivePower=5000  InductivePower=0  CapacitivePower=0  Measurements=None  LoadType=constant Z
  in_a : PMIOPort  Port=1  Side=Left
  in_b : PMIOPort  Port=2  Side=Left
  in_c : PMIOPort  Port=3  Side=Left
  out_a : PMIOPort  Port=4  Side=Right
  out_b : PMIOPort  Port=5  Side=Right
  out_c : PMIOPort  Port=6  Side=Right
  Vabc : Outport
  Iabc : Outport  Port=2
  wires:
  GLC control/1 -> Contactor/1(com)
  P.O.R  and CTA/1 -> Vabc/1
  P.O.R  and CTA/2 -> Iabc/1
  connections:
  in_a/RConn1 -- P.O.R  and CTA/LConn1 -- parasitic resistive load/LConn1
  in_b/RConn1 -- P.O.R  and CTA/LConn2 -- parasitic resistive load/LConn2
  in_c/RConn1 -- P.O.R  and CTA/LConn3 -- parasitic resistive load/LConn3
  P.O.R  and CTA/RConn1 -- Contactor/LConn1
  P.O.R  and CTA/RConn2 -- Contactor/LConn2
  P.O.R  and CTA/RConn3 -- Contactor/LConn3
  Contactor/RConn1 -- out_a/RConn1
  out_b/RConn1 -- Contactor/RConn2
  Contactor/RConn3 -- out_c/RConn1

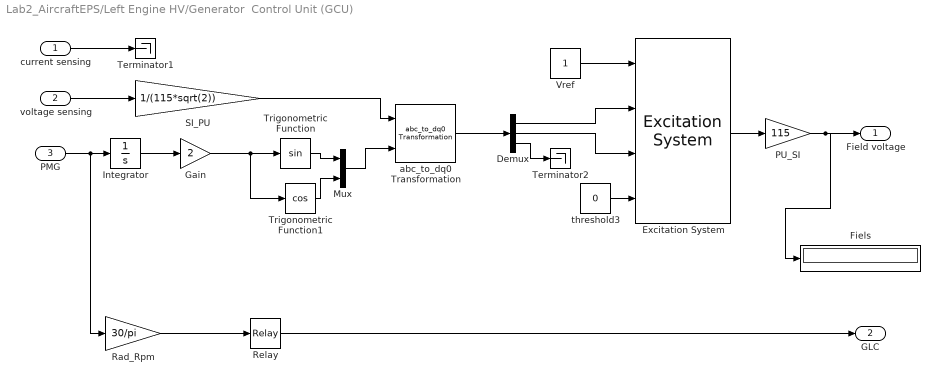
== system Lab2_AircraftEPS/Left Engine HV/Generator  Control Unit (GCU) ==
  current sensing : Inport
  voltage sensing : Inport  Port=2
  PMG : Inport  Port=3
  Demux : Demux  Outputs=3
  Excitation System : sps_avr/Excitation System   tr=20e-3  reg=[ 300, 0.001 ]  exc=[ 1, 0 ]  tgr=[ 0, 0 ]  damp=[ 0.001, 0.1 ]  sat=[ 0, 0 ]  lim=[ -2, 2, 0 ]  v0=[1 0]
  Fiels : Display
      settings: SampleTime=1e-2
  Gain : Gain  Gain=2
  Integrator : Integrator
  Mux : Mux  Inputs=2
  PU_SI : Gain  Gain=115
  Rad_Rpm : Gain  Gain=30/pi
  Relay : Relay  OnSwitchValue=9000  OffSwitchValue=8900
  SI_PU : Gain  Gain=1/(115*sqrt(2))
  Terminator1 : Terminator
  Terminator2 : Terminator
  Trigonometric Function : Trigonometry
  Trigonometric Function1 : Trigonometry  Operator=cos
  Vref : Constant
  abc_to_dq0 Transformation : powerlib_extras/Measurements/abc_to_dq0 Transformation
  threshold3 : Constant  Value=0
  Field voltage : Outport
  GLC : Outport  Port=2
  wires:
  Relay/1 -> GLC/1
  Demux/3 -> Terminator2/1
  current sensing/1 -> Terminator1/1
  threshold3/1 -> Excitation System/4
  Vref/1 -> Excitation System/1
  Rad_Rpm/1 -> Relay/1
  PU_SI/1 -> Field voltage/1, Fiels/1
  Excitation System/1 -> PU_SI/1
  SI_PU/1 -> abc_to_dq0 Transformation/1
  Demux/2 -> Excitation System/3
  Demux/1 -> Excitation System/2
  abc_to_dq0 Transformation/1 -> Demux/1
  Mux/1 -> abc_to_dq0 Transformation/2
  Trigonometric Function1/1 -> Mux/2
  Trigonometric Function/1 -> Mux/1
  Gain/1 -> Trigonometric Function1/1, Trigonometric Function/1
  Integrator/1 -> Gain/1
  voltage sensing/1 -> SI_PU/1
  PMG/1 -> Rad_Rpm/1, Integrator/1

== system Lab2_AircraftEPS/Left Engine HV/Mechanical engine (turbine) ==
  Demux : Demux  Tag=STV Demux  Outputs=1
  FromWs : FromWorkspace  Tag=STV FromWs  VariableName=tuvar  SampleTime=0  SigBuilderData=DataTag4  VnvData=DataTag5
      SigBuilderData=|
      | common.afterFinalStr = 'Extrapolate'
      | common.sampleTime = 0
      | dataSet.timeRange = [0 10]
      | dataSet.name = 'Group 1'
      | sbobj.Groups.Name = 'Group 1'
      | sbobj.Groups.Signals.Name = 'Signal 1'
      | sbobj.Groups.Signals.XData = [0 0.2 0.4 0.5 1 2 3 4.5 6 10]
      | sbobj.Groups.Signals.YData = [15000 15000 15000 15000 15000 15000 15000 15000 15000 15000]
  Signal 1 : Outport  Tag=STV Outport
  wires:
  FromWs/1 -> Demux/1
  Demux/1 -> Signal 1/1

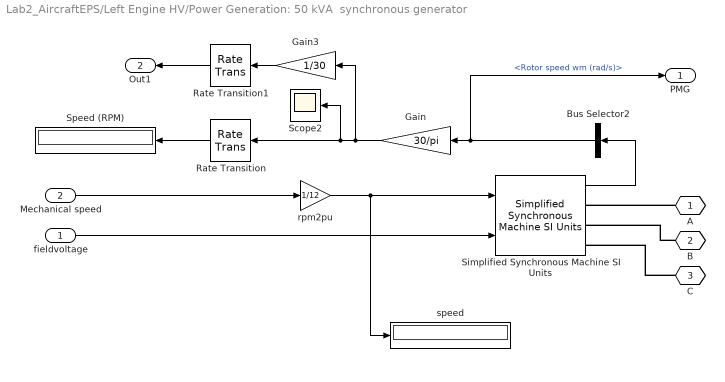
== system Lab2_AircraftEPS/Left Engine HV/Power Generation: 50 kVA  synchronous generator ==
  fieldvoltage : Inport
  Mechanical speed : Inport  Port=2
  Bus Selector2 : BusSelector  OutputSignals=Rotor speed wm (rad/s)
  Gain : Gain  Gain=30/pi
  Gain3 : Gain  Gain=1/30
  Rate Transition : RateTransition  OutPortSampleTimeOpt=Inherit  OutPortSampleTime=Ts
  Rate Transition1 : RateTransition  OutPortSampleTimeOpt=Inherit  OutPortSampleTime=Ts
  Scope2 : Scope
      settings: TimeRange=1  YMin=13545  YMax=13575  SaveName=ScopeData3  Decimation=100  SampleTime=1e-3
  Simplified Synchronous Machine SI Units : powerlib/Machines/Simplified Synchronous Machine SI Units  ConnectionType=3-wire Y  MechanicalLoad=Speed w  NominalParameters=[50e3 115 400]  Mechanical=[0.02 0 2]  InternalRL="[0.0204  0.08104e-3]"  InitialConditions=[-99,0 0,0,0 0,0,0]  Units=1  LoadFlowParameters=[1 0 0 0 0]  TsPowergui=0  TsBlock=-1  BusType=PV  Pref=0  Qref=0  Qmin=-inf  Qmax=+inf  PLF=0  QLF=0
  Speed (RPM) : Display
      settings: SampleTime=1e-2
  rpm2pu : Gain  Gain=1/12
  speed : Display
      settings: SampleTime=1e-2
  A : PMIOPort  Tag=PMCPort  Port=1  Side=Right
  B : PMIOPort  Tag=PMCPort  Port=2  Side=Right
  C : PMIOPort  Tag=PMCPort  Port=3  Side=Right
  PMG : Outport
  Out1 : Outport  Port=2
  wires:
  Simplified Synchronous Machine SI Units/1 -> Bus Selector2/1
  fieldvoltage/1 -> Simplified Synchronous Machine SI Units/2
  Bus Selector2/1 -> Gain/1, PMG/1  "<Rotor speed wm (rad/s)>"
  Gain/1 -> Gain3/1, Scope2/1, Rate Transition/1
  Gain3/1 -> Rate Transition1/1
  Mechanical speed/1 -> rpm2pu/1
  rpm2pu/1 -> Simplified Synchronous Machine SI Units/1, speed/1
  Rate Transition/1 -> Speed (RPM)/1
  Rate Transition1/1 -> Out1/1
  connections:
  A/RConn1 -- Simplified Synchronous Machine SI Units/RConn1
  B/RConn1 -- Simplified Synchronous Machine SI Units/RConn2
  C/RConn1 -- Simplified Synchronous Machine SI Units/RConn3

== system Lab2_AircraftEPS/Left Engine HV/Sensor ==
  Three Phase  Measurement : powerlib/Measurements/Three-Phase V-I Measurement  VoltageMeasurement=phase-to-phase  SetLabelV=off  LabelV=Vabc  Vpu=off  VpuLL=off  CurrentMeasurement=yes  SetLabelI=off  LabelI=Iabc  Ipu=off  Pbase=100e6  Vbase=500e3  OutputType=Complex  PhasorSimulation=off  PSBequivalent=0
  parasitic  load : powerlib/Elements/Three-Phase Series RLC Load  LConnTagsString=A|B|C  Configuration=Y (grounded)  NominalVoltage=115  NominalFrequency=400  ActivePower=5000  InductivePower=0  CapacitivePower=0  Measurements=None  LoadType=constant Z
  A : PMIOPort  Port=1  Side=Left
  B : PMIOPort  Port=2  Side=Left
  a : PMIOPort  Port=3  Side=Right
  b : PMIOPort  Port=4  Side=Right
  C : PMIOPort  Port=5  Side=Left
  c : PMIOPort  Port=6  Side=Right
  Vabc : Outport
  Iabc : Outport  Port=2
  wires:
  Three Phase  Measurement/1 -> Vabc/1
  Three Phase  Measurement/2 -> Iabc/1
  connections:
  A/RConn1 -- Three Phase  Measurement/LConn1 -- parasitic  load/LConn1
  B/RConn1 -- Three Phase  Measurement/LConn2 -- parasitic  load/LConn2
  C/RConn1 -- Three Phase  Measurement/LConn3 -- parasitic  load/LConn3
  a/RConn1 -- Three Phase  Measurement/RConn1
  b/RConn1 -- Three Phase  Measurement/RConn2
  c/RConn1 -- Three Phase  Measurement/RConn3

== system Lab2_AircraftEPS/Right Engine HV/Fault Contactor ==
  Fault : Inport
  In1 : Inport  Port=2
  Constant : Constant  Value=0
  Switch : Switch  Threshold=0.5
  out : Outport
  wires:
  Fault/1 -> Switch/2
  Constant/1 -> Switch/3
  In1/1 -> Switch/1
  Switch/1 -> out/1

== system Lab2_AircraftEPS/Right Engine HV/Feedback measurements &  main contactor ==
  note: Primary Distribution
  GLC control : Inport
  Contactor : Subsystem
  P.O.R  and CTA : powerlib/Measurements/Three-Phase V-I Measurement  VoltageMeasurement=phase-to-phase  SetLabelV=off  LabelV=Vabc  Vpu=off  VpuLL=off  CurrentMeasurement=yes  SetLabelI=off  LabelI=Iabc  Ipu=off  Pbase=100e6  Vbase=500e3  OutputType=Complex  PhasorSimulation=off  PSBequivalent=0
  parasitic resistive load : powerlib/Elements/Three-Phase Series RLC Load  LConnTagsString=A|B|C  Configuration=Y (grounded)  NominalVoltage=115  NominalFrequency=400  ActivePower=5000  InductivePower=0  CapacitivePower=0  Measurements=None  LoadType=constant Z
  in_a : PMIOPort  Port=1  Side=Left
  in_b : PMIOPort  Port=2  Side=Left
  in_c : PMIOPort  Port=3  Side=Left
  out_a : PMIOPort  Port=4  Side=Right
  out_b : PMIOPort  Port=5  Side=Right
  out_c : PMIOPort  Port=6  Side=Right
  Vabc : Outport
  Iabc : Outport  Port=2
  wires:
  GLC control/1 -> Contactor/1(com)
  P.O.R  and CTA/1 -> Vabc/1
  P.O.R  and CTA/2 -> Iabc/1
  connections:
  in_a/RConn1 -- P.O.R  and CTA/LConn1 -- parasitic resistive load/LConn1
  in_b/RConn1 -- P.O.R  and CTA/LConn2 -- parasitic resistive load/LConn2
  in_c/RConn1 -- P.O.R  and CTA/LConn3 -- parasitic resistive load/LConn3
  P.O.R  and CTA/RConn1 -- Contactor/LConn1
  P.O.R  and CTA/RConn2 -- Contactor/LConn2
  P.O.R  and CTA/RConn3 -- Contactor/LConn3
  Contactor/RConn1 -- out_a/RConn1
  out_b/RConn1 -- Contactor/RConn2
  Contactor/RConn3 -- out_c/RConn1

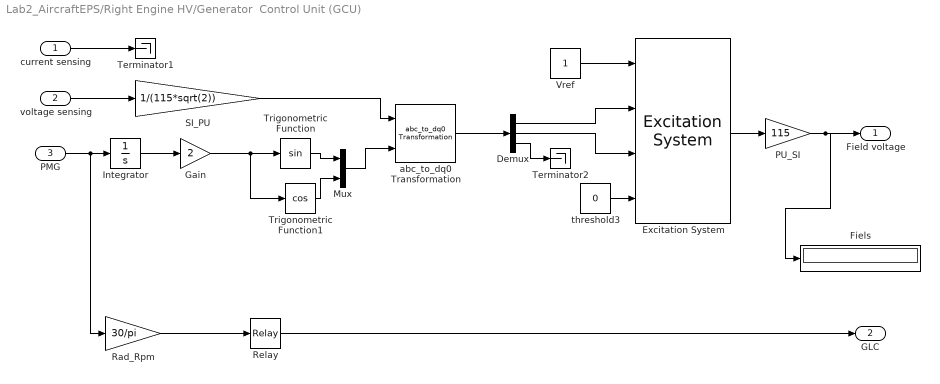
== system Lab2_AircraftEPS/Right Engine HV/Generator  Control Unit (GCU) ==
  current sensing : Inport
  voltage sensing : Inport  Port=2
  PMG : Inport  Port=3
  Demux : Demux  Outputs=3
  Excitation System : sps_avr/Excitation System   tr=20e-3  reg=[ 300, 0.001 ]  exc=[ 1, 0 ]  tgr=[ 0, 0 ]  damp=[ 0.001, 0.1 ]  sat=[ 0, 0 ]  lim=[ -2, 2, 0 ]  v0=[1 0]
  Fiels : Display
      settings: SampleTime=1e-2
  Gain : Gain  Gain=2
  Integrator : Integrator
  Mux : Mux  Inputs=2
  PU_SI : Gain  Gain=115
  Rad_Rpm : Gain  Gain=30/pi
  Relay : Relay  OnSwitchValue=9000  OffSwitchValue=8900
  SI_PU : Gain  Gain=1/(115*sqrt(2))
  Terminator1 : Terminator
  Terminator2 : Terminator
  Trigonometric Function : Trigonometry
  Trigonometric Function1 : Trigonometry  Operator=cos
  Vref : Constant
  abc_to_dq0 Transformation : powerlib_extras/Measurements/abc_to_dq0 Transformation
  threshold3 : Constant  Value=0
  Field voltage : Outport
  GLC : Outport  Port=2
  wires:
  Relay/1 -> GLC/1
  Demux/3 -> Terminator2/1
  current sensing/1 -> Terminator1/1
  threshold3/1 -> Excitation System/4
  Vref/1 -> Excitation System/1
  Rad_Rpm/1 -> Relay/1
  PU_SI/1 -> Field voltage/1, Fiels/1
  Excitation System/1 -> PU_SI/1
  SI_PU/1 -> abc_to_dq0 Transformation/1
  Demux/2 -> Excitation System/3
  Demux/1 -> Excitation System/2
  abc_to_dq0 Transformation/1 -> Demux/1
  Mux/1 -> abc_to_dq0 Transformation/2
  Trigonometric Function1/1 -> Mux/2
  Trigonometric Function/1 -> Mux/1
  Gain/1 -> Trigonometric Function1/1, Trigonometric Function/1
  Integrator/1 -> Gain/1
  voltage sensing/1 -> SI_PU/1
  PMG/1 -> Rad_Rpm/1, Integrator/1

== system Lab2_AircraftEPS/Right Engine HV/Mechanical engine (turbine) ==
  Demux : Demux  Tag=STV Demux  Outputs=1
  FromWs : FromWorkspace  Tag=STV FromWs  VariableName=tuvar  SampleTime=0  SigBuilderData=DataTag6  VnvData=DataTag7
      SigBuilderData=|
      | common.afterFinalStr = 'Extrapolate'
      | common.sampleTime = 0
      | dataSet.timeRange = [0 10]
      | dataSet.name = 'Group 1'
      | sbobj.Groups.Name = 'Group 1'
      | sbobj.Groups.Signals.Name = 'Signal 1'
      | sbobj.Groups.Signals.XData = [0 0.2 0.4 0.5 1 2 3 4.5 6 10]
      | sbobj.Groups.Signals.YData = [15000 15000 15000 15000 15000 15000 15000 15000 15000 15000]
  Signal 1 : Outport  Tag=STV Outport
  wires:
  FromWs/1 -> Demux/1
  Demux/1 -> Signal 1/1

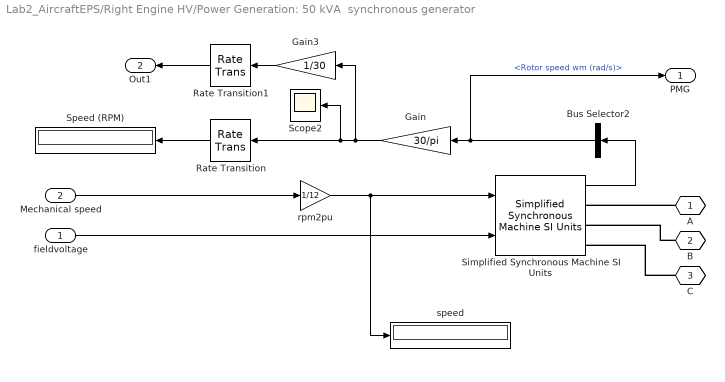
== system Lab2_AircraftEPS/Right Engine HV/Power Generation: 50 kVA  synchronous generator ==
  fieldvoltage : Inport
  Mechanical speed : Inport  Port=2
  Bus Selector2 : BusSelector  OutputSignals=Rotor speed wm (rad/s)
  Gain : Gain  Gain=30/pi
  Gain3 : Gain  Gain=1/30
  Rate Transition : RateTransition  OutPortSampleTimeOpt=Inherit  OutPortSampleTime=Ts
  Rate Transition1 : RateTransition  OutPortSampleTimeOpt=Inherit  OutPortSampleTime=Ts
  Scope2 : Scope
      settings: TimeRange=1  YMin=13545  YMax=13575  SaveName=ScopeData3  Decimation=100  SampleTime=1e-3
  Simplified Synchronous Machine SI Units : powerlib/Machines/Simplified Synchronous Machine SI Units  ConnectionType=3-wire Y  MechanicalLoad=Speed w  NominalParameters=[50e3 115 400]  Mechanical=[0.02 0 2]  InternalRL="[0.0204  0.08104e-3]"  InitialConditions=[-99,0 0,0,0 0,0,0]  Units=1  LoadFlowParameters=[1 0 0 0 0]  TsPowergui=0  TsBlock=-1  BusType=PV  Pref=0  Qref=0  Qmin=-inf  Qmax=+inf  PLF=0  QLF=0
  Speed (RPM) : Display
      settings: SampleTime=1e-2
  rpm2pu : Gain  Gain=1/12
  speed : Display
      settings: SampleTime=1e-2
  A : PMIOPort  Tag=PMCPort  Port=1  Side=Right
  B : PMIOPort  Tag=PMCPort  Port=2  Side=Right
  C : PMIOPort  Tag=PMCPort  Port=3  Side=Right
  PMG : Outport
  Out1 : Outport  Port=2
  wires:
  Simplified Synchronous Machine SI Units/1 -> Bus Selector2/1
  fieldvoltage/1 -> Simplified Synchronous Machine SI Units/2
  Bus Selector2/1 -> Gain/1, PMG/1  "<Rotor speed wm (rad/s)>"
  Gain/1 -> Gain3/1, Scope2/1, Rate Transition/1
  Gain3/1 -> Rate Transition1/1
  Mechanical speed/1 -> rpm2pu/1
  rpm2pu/1 -> Simplified Synchronous Machine SI Units/1, speed/1
  Rate Transition/1 -> Speed (RPM)/1
  Rate Transition1/1 -> Out1/1
  connections:
  A/RConn1 -- Simplified Synchronous Machine SI Units/RConn1
  B/RConn1 -- Simplified Synchronous Machine SI Units/RConn2
  C/RConn1 -- Simplified Synchronous Machine SI Units/RConn3

== system Lab2_AircraftEPS/Right Engine HV/Sensor ==
  Three Phase  Measurement : powerlib/Measurements/Three-Phase V-I Measurement  VoltageMeasurement=phase-to-phase  SetLabelV=off  LabelV=Vabc  Vpu=off  VpuLL=off  CurrentMeasurement=yes  SetLabelI=off  LabelI=Iabc  Ipu=off  Pbase=100e6  Vbase=500e3  OutputType=Complex  PhasorSimulation=off  PSBequivalent=0
  parasitic  load : powerlib/Elements/Three-Phase Series RLC Load  LConnTagsString=A|B|C  Configuration=Y (grounded)  NominalVoltage=115  NominalFrequency=400  ActivePower=5000  InductivePower=0  CapacitivePower=0  Measurements=None  LoadType=constant Z
  A : PMIOPort  Port=1  Side=Left
  B : PMIOPort  Port=2  Side=Left
  a : PMIOPort  Port=3  Side=Right
  b : PMIOPort  Port=4  Side=Right
  C : PMIOPort  Port=5  Side=Left
  c : PMIOPort  Port=6  Side=Right
  Vabc : Outport
  Iabc : Outport  Port=2
  wires:
  Three Phase  Measurement/1 -> Vabc/1
  Three Phase  Measurement/2 -> Iabc/1
  connections:
  A/RConn1 -- Three Phase  Measurement/LConn1 -- parasitic  load/LConn1
  B/RConn1 -- Three Phase  Measurement/LConn2 -- parasitic  load/LConn2
  C/RConn1 -- Three Phase  Measurement/LConn3 -- parasitic  load/LConn3
  a/RConn1 -- Three Phase  Measurement/RConn1
  b/RConn1 -- Three Phase  Measurement/RConn2
  c/RConn1 -- Three Phase  Measurement/RConn3

== system Lab2_AircraftEPS/APU1/Feedback measurements &  main contactor/Contactor ==
  com : Inport
  Ideal Switch : powerlib/Power Electronics/Ideal Switch  Ron=0.001  Lon=0  IC=0  Rs=1e3  Cs=inf  Measurements=off
  Ideal Switch1 : powerlib/Power Electronics/Ideal Switch  Ron=0.001  Lon=0  IC=0  Rs=1e3  Cs=inf  Measurements=off
  Ideal Switch2 : powerlib/Power Electronics/Ideal Switch  Ron=0.001  Lon=0  IC=0  Rs=1e3  Cs=inf  Measurements=off
  A : PMIOPort  Port=1  Side=Left
  a : PMIOPort  Port=2  Side=Right
  B : PMIOPort  Port=3  Side=Left
  b : PMIOPort  Port=4  Side=Right
  C : PMIOPort  Port=5  Side=Left
  c : PMIOPort  Port=6  Side=Right
  wires:
  com/1 -> Ideal Switch1/1, Ideal Switch2/1, Ideal Switch/1
  connections:
  c/RConn1 -- Ideal Switch2/RConn1
  C/RConn1 -- Ideal Switch2/LConn1
  b/RConn1 -- Ideal Switch1/RConn1
  B/RConn1 -- Ideal Switch1/LConn1
  a/RConn1 -- Ideal Switch/RConn1
  A/RConn1 -- Ideal Switch/LConn1

== system Lab2_AircraftEPS/APU2/Feedback measurements &  main contactor/Contactor ==
  com : Inport
  Ideal Switch : powerlib/Power Electronics/Ideal Switch  Ron=0.001  Lon=0  IC=0  Rs=1e3  Cs=inf  Measurements=off
  Ideal Switch1 : powerlib/Power Electronics/Ideal Switch  Ron=0.001  Lon=0  IC=0  Rs=1e3  Cs=inf  Measurements=off
  Ideal Switch2 : powerlib/Power Electronics/Ideal Switch  Ron=0.001  Lon=0  IC=0  Rs=1e3  Cs=inf  Measurements=off
  A : PMIOPort  Port=1  Side=Left
  a : PMIOPort  Port=2  Side=Right
  B : PMIOPort  Port=3  Side=Left
  b : PMIOPort  Port=4  Side=Right
  C : PMIOPort  Port=5  Side=Left
  c : PMIOPort  Port=6  Side=Right
  wires:
  com/1 -> Ideal Switch1/1, Ideal Switch2/1, Ideal Switch/1
  connections:
  c/RConn1 -- Ideal Switch2/RConn1
  C/RConn1 -- Ideal Switch2/LConn1
  b/RConn1 -- Ideal Switch1/RConn1
  B/RConn1 -- Ideal Switch1/LConn1
  a/RConn1 -- Ideal Switch/RConn1
  A/RConn1 -- Ideal Switch/LConn1

== system Lab2_AircraftEPS/Left Engine HV/Feedback measurements &  main contactor/Contactor ==
  com : Inport
  Ideal Switch : powerlib/Power Electronics/Ideal Switch  Ron=0.001  Lon=0  IC=0  Rs=1e3  Cs=inf  Measurements=off
  Ideal Switch1 : powerlib/Power Electronics/Ideal Switch  Ron=0.001  Lon=0  IC=0  Rs=1e3  Cs=inf  Measurements=off
  Ideal Switch2 : powerlib/Power Electronics/Ideal Switch  Ron=0.001  Lon=0  IC=0  Rs=1e3  Cs=inf  Measurements=off
  A : PMIOPort  Port=1  Side=Left
  a : PMIOPort  Port=2  Side=Right
  B : PMIOPort  Port=3  Side=Left
  b : PMIOPort  Port=4  Side=Right
  C : PMIOPort  Port=5  Side=Left
  c : PMIOPort  Port=6  Side=Right
  wires:
  com/1 -> Ideal Switch1/1, Ideal Switch2/1, Ideal Switch/1
  connections:
  c/RConn1 -- Ideal Switch2/RConn1
  C/RConn1 -- Ideal Switch2/LConn1
  b/RConn1 -- Ideal Switch1/RConn1
  B/RConn1 -- Ideal Switch1/LConn1
  a/RConn1 -- Ideal Switch/RConn1
  A/RConn1 -- Ideal Switch/LConn1

== system Lab2_AircraftEPS/Right Engine HV/Feedback measurements &  main contactor/Contactor ==
  com : Inport
  Ideal Switch : powerlib/Power Electronics/Ideal Switch  Ron=0.001  Lon=0  IC=0  Rs=1e3  Cs=inf  Measurements=off
  Ideal Switch1 : powerlib/Power Electronics/Ideal Switch  Ron=0.001  Lon=0  IC=0  Rs=1e3  Cs=inf  Measurements=off
  Ideal Switch2 : powerlib/Power Electronics/Ideal Switch  Ron=0.001  Lon=0  IC=0  Rs=1e3  Cs=inf  Measurements=off
  A : PMIOPort  Port=1  Side=Left
  a : PMIOPort  Port=2  Side=Right
  B : PMIOPort  Port=3  Side=Left
  b : PMIOPort  Port=4  Side=Right
  C : PMIOPort  Port=5  Side=Left
  c : PMIOPort  Port=6  Side=Right
  wires:
  com/1 -> Ideal Switch1/1, Ideal Switch2/1, Ideal Switch/1
  connections:
  c/RConn1 -- Ideal Switch2/RConn1
  C/RConn1 -- Ideal Switch2/LConn1
  b/RConn1 -- Ideal Switch1/RConn1
  B/RConn1 -- Ideal Switch1/LConn1
  a/RConn1 -- Ideal Switch/RConn1
  A/RConn1 -- Ideal Switch/LConn1

== matlab function BPCU/MATLAB Function ==
  data: in_bus input double; contactors output double
% for a more verbose explanation of the logic, see:
% ee249_lab2/BPCU_pseudocode/BPCU_pseudocode_withX.m

function contactors  = BPCU_core(in_bus)
    GL = in_bus(1);
    AL = in_bus(2);
    AR = in_bus(3);
    GR = in_bus(4);
    
    c = zeros([1 6]); %simulink wants me to preallocate
    if GL && GR
        c = [1 0 0 1 0 0]; %GL power left, GR power right
    elseif ~GL && GR
        if AL
            c = [0 1 0 1 1 0]; %GL off, GR power right, AL power left 
        elseif AR
            c = [0 0 1 1 1 0]; %GL off, GR power right, AR power left
        else
            c = [0 0 0 1 1 1]; %GR power whole plane, everything else off
        end
    elseif GL && ~GR
        if AR
            c = [1 0 1 0 0 1]; %GR off, GL power left, AR power right
        elseif AL
            c = [1 1 0 0 0 1]; %GR off, GL power left, AL power right
        else
            c = [1 0 0 0 1 1]; %GL power whole plane, everything else off
        end
    elseif ~GL && ~GR
        %it's arbitrary whether to use AL or AR in this case
        if AR
            c = [0 0 1 0 1 1]; %GL off, GR off, AR power whole plane
        elseif AL
            c = [0 1 0 0 1 1]; %GL off, GR off, AL power whole plane
        else
            c = [0 0 0 0 0 0]; %all generators are broken ... good luck with that.
        end
    end

    %append on/off status for the B7-B12. B7,B8,B9,B10 are always on, and B11,B12 are always off
    contactors = [c 1 1 1 1 0 0];
